simulink library "cordic_rotation_mode"  (R2018b)
settings: Solver=VariableStepAuto  StartTime=0.0  StopTime=10.0  RelTol=1e-3
undefined symbols (not defined in the file or in its folder): nIters
settings Model: Creator=jimjoy  LastModifiedBy=tbryan
settings DataIOCC: ReturnWorkspaceOutputs=on

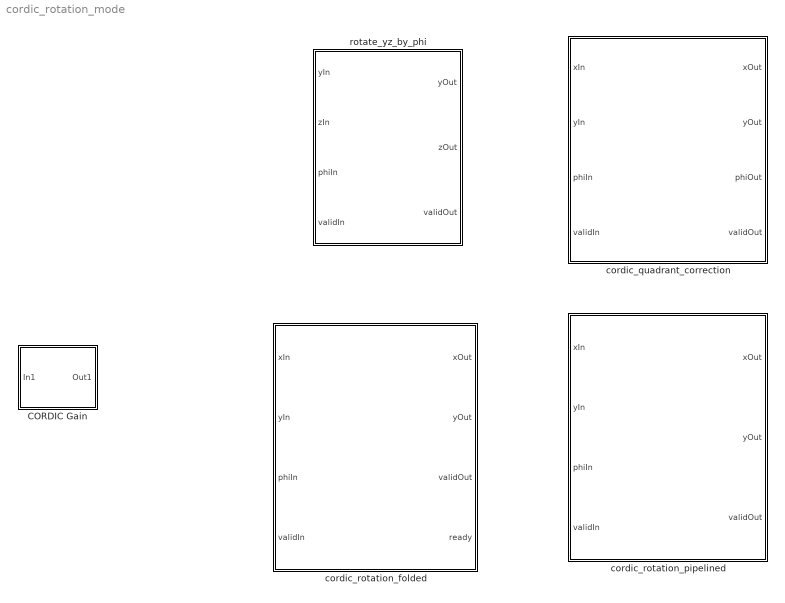
== system cordic_rotation_mode ==
  CORDIC Gain : Subsystem  mask{nIters=nIters}
      mask prompts: nIters "Number of CORDIC Iterations"
  cordic_quadrant_correction : MATLAB Function  TreatAsAtomicUnit=on
  cordic_rotation_folded : MATLAB Function  TreatAsAtomicUnit=on  mask{nIters=nIters}
      mask prompts: nIters "Number of CORDIC Iterations"
  cordic_rotation_pipelined : MATLAB Function  TreatAsAtomicUnit=on
  rotate_yz_by_phi : MATLAB Function  TreatAsAtomicUnit=on  mask{nIters=nIters}
      mask prompts: nIters "Number of CORDIC Iterations"

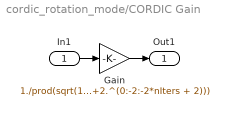
== system cordic_rotation_mode/CORDIC Gain ==
  In1 : Inport
  Gain : Gain  Gain=1./prod(sqrt(1+2.^(0:-2:-2*nIters + 2)))  OutDataTypeStr=Inherit: Same as input
  Out1 : Outport
  wires:
  Gain/1 -> Out1/1
  In1/1 -> Gain/1

== matlab function cordic_rotation_mode/cordic_quadrant_correction ==
  settings: fimath=hdlfimath
  data: xIn input; xOut output; yIn input; phiIn input; validIn input boolean; yOut output; phiOut output; validOut output
function [xOut, yOut, phiOut, validOut] = cordic_quadrant_correction(xIn, yIn, phiIn, validIn)
    
    % Copyright 2018 The MathWorks, Inc.
    %#codegen
   
    persistent xReg yReg phiReg validReg
    
    T = constructTypesTable(xIn, yIn, phiIn, validIn);
    
    if isempty(xReg)
       xReg = cast(0,'like',T.x);
       yReg = cast(0,'like',T.y);
       phiReg = cast(0,'like',T.phi);
       validReg = cast(0,'like',T.validIn);
    end
    
    xOut = xReg;
    yOut = yReg;
    phiOut = phiReg;
    validOut = validReg;
   

    [xReg, yReg, phiReg] = cordicQuadrantCorrectionKernel(xIn, yIn, phiIn, T);
    validReg = cast(validIn, 'like', T.validIn);
    
end

function T = constructTypesTable(x, y ,phi, validIn)
    % This convenience function constructs the types table for the
    % cordic quadrant correction. It also provides some top level
    % assertions that are evaluated at compile time.
    coder.inline('always');
    if isfloat(x)
        assert(isfloat(y),'X and Y must Both be floating poitn values')
        isHDL = coder.target('HDL');
        assert(~isHDL,'Floating-point is not supported for this function in HDL Code Generation');
        T.x = cast([],'like',x);
        T.y = cast([],'like',y);
    elseif isfi(x)
        assert(isfi(y), 'X and Y must both be fi objects');
        assert(isscaledtype(x) && isscaledtype(y),'X and Y must be scaled types');
        % Assert that the wordlength and fraction length are equal
        assert((x.WordLength == y.WordLength) && ...
                              (x.FractionLength == y.FractionLength),'X and Y must have the same word and fraction lengths');
        wl = max(8, x.WordLength);
        fl = min(wl - 3, x.FractionLength);
        F = hdlfimath();
        T.x = fi([],1,wl,fl,F);
        T.y = fi([],1,wl,fl,F);
    else
       assert(false,'Type not supported');
    end
    
    assert(isfloat(phi) || (isfi(phi) && isscaledtype(phi)), 'phi must be either floating point or a scaled fi type');
    T.phi = cast([],'like',phi);
    
    assert(islogical(validIn) || (isfi(validIn) && isboolean(validIn)),'validIn must be logical');
    T.validIn = cast([],'like',validIn);
end

function [xOut, yOut, phiOut] = cordicQuadrantCorrectionKernel(x, y, phi, T)
    coder.inline('always');
    xOut = cast(x,'like',T.x);
    yOut = cast(y,'like',T.y);
    phiOut = cast(phi,'like',T.phi);
    if (phi > coder.const(cast(pi/2,'like', T.phi))) && ...
            (phi < coder.const(cast(1.5*pi,'like', T.phi)))
        phiOut(:) = phi - cast(pi,'like', T.phi);
        xOut(:) = -x;
        yOut(:) = -y;
    elseif (phi > coder.const(cast(1.5*pi,'like', T.phi)))
        phiOut(:) = phi - cast(2*pi,'like', T.phi);
        xOut(:) = x;
        yOut(:) = y;
    elseif (phi < cast(-0.5*pi,'like', T.phi))
        phiOut(:) = phi + cast(pi,'like',T.phi);
        xOut(:) = -x;
        yOut(:) = -y;
    end
end

== matlab function cordic_rotation_mode/rotate_yz_by_phi ==
  settings: fimath=hdlfimath
  data: yIn input; zIn input; yOut output; zOut output; phiIn input; validIn input; validOut output; nIters parameter
function [yOut, zOut, validOut] = rotate_by_phi(yIn, zIn, phiIn, validIn, nIters)
    %#codegen
    
    %Copyright 2018 The MathWorks, Inc.
    
    persistent yReg zReg validReg phiReg
    
    yNumericTypeInternal = numerictype(1,yIn.WordLength + 3, yIn.FractionLength + 3);
    zNumericTypeInternal = numerictype(1,zIn.WordLength + 3, zIn.FractionLength + 3);
    phiNumericTypeInternal = numerictype(1,zIn.WordLength+3, zIn.FractionLength + 3);
    
    if isempty(yReg)
        yReg = fi(zeros(1,nIters+2), yNumericTypeInternal);
        zReg = fi(zeros(1,nIters+2), zNumericTypeInternal);
        phiReg = fi(zeros(1,nIters+2), phiNumericTypeInternal);
        validReg = false(1,nIters+2);
    end
    
    yOut = cast(yReg(end),'like',yIn);
    zOut = cast(zReg(end),'like',zIn);
    validOut = validReg(end);
    coder.unroll
    for ii = nIters+2:-1:1
        if ii == 1
            [yReg(ii), zReg(ii), phiReg(ii), validReg(ii)] = ...
                readInputs(yIn, zIn, phiIn, validIn);
        elseif ii == 2
            validReg(ii) = validReg(ii - 1);
            [yReg(ii), zReg(ii), phiReg(ii)] = ...
                cordicQuadrantCorrection(yReg(ii-1), zReg(ii - 1), phiReg(ii-1));
        else
            validReg(ii) = validReg(ii - 1);
            [yReg(ii), zReg(ii), phiReg(ii)] = ...
                cordicRotationKernel(yReg(ii-1), zReg(ii - 1), phiReg(ii - 1),...
                ii, nIters);
        end
    end
    
end

function [y, z, phi, valid] = readInputs(yIn, zIn, phiIn, validIn)
    y = yIn;
    z = zIn;
    phi = phiIn;
    valid = validIn;
end

function [yOut, zOut, phiOut] = cordicQuadrantCorrection(y, z, phi)
    yOut = y;
    zOut = z;
    phiOut = phi;
    if (phi > coder.const(cast(pi/2,'like',phi))) && ...
            (phi < coder.const(cast(1.5*pi,'like',phi)))
        phiOut(:) = phi - cast(pi,'like',phi);
        yOut(:) = -y;
        zOut(:) = -z;
    elseif (phi > coder.const(cast(1.5*pi,'like',phi)))
        phiOut(:) = phi - cast(2*pi,'like',phi);
        yOut(:) = y;
        zOut(:) = z;
    end
end

function [yOut, zOut, phiOut] = cordicRotationKernel(y, z, phi, iterNum, numIters)
    angleTable = coder.const(getAngleTable(numIters,phi));
    y0 = bitsra(y,iterNum - 3);
    z0 = bitsra(z,iterNum - 3);
    yOut = y;
    zOut = z;
    phiOut = phi;
    if phi > 0
        % Rotate in the positive direction
        yOut(:) = y - z0;
        zOut(:) = z + y0;
        phiOut(:) = phi - angleTable(iterNum - 2);
    else
        % Rotate in the negative direction
        yOut(:) = y + z0;
        zOut(:) = z - y0;
        phiOut(:) = phi + angleTable(iterNum - 2);
    end
end

function angleTable = getAngleTable(numIters, T)
    angleTable = cast(atan(2.^(0:-1:-numIters + 1)),'like',T);
end

== matlab function cordic_rotation_mode/cordic_rotation_pipelined ==
  settings: fimath=hdlfimath
  data: xIn input; xOut output; yIn input; phiIn input; validIn input; yOut output; validOut output; nIters parameter
function [xOut, yOut, validOut] = cordic_rotation_pipelined(xIn, yIn, phiIn, validIn, nIters)
   
    % Copyright 2018 The MathWorks, Inc.
    
    %#codegen
    
    persistent xReg yReg validReg phiReg
    
    T = getTypesTable(xIn, yIn, phiIn, validIn);
    
    if isempty(xReg)
       xReg = zeros(nIters + 1,1,'like',T.x);
       yReg = zeros(nIters + 1,1,'like',T.y);
       phiReg = zeros(nIters + 1,1,'like',T.phi);
       validReg = zeros(nIters + 1,1,'like',T.validIn);
    end
    
    xOut = xReg(end);
    yOut = yReg(end);
    validOut = validReg(end);
    
    validReg(:) = [validIn; validReg(1:end-1)];
    [xReg(2:end), yReg(2:end), phiReg(2:end)] = ...
        cordicRotationKernel(xReg(1:end-1), yReg(1:end-1), phiReg(1:end-1), nIters, T);
    xReg(1) = xIn;
    yReg(1) = yIn;
    phiReg(1) = phiIn;
    
end

function T = getTypesTable(x, y, phi, validIn)
    % This convenience function constructs the types table for the
    % cordic quadrant correction. It also provides some top level
    % assertions that are evaluated at compile time.
    coder.inline('always');
    if isfloat(x)
        assert(isfloat(y),'X and Y must Both be floating poitn values')
        isHDL = coder.target('HDL');
        assert(~isHDL,'Floating-point is not supported for this function in HDL Code Generation');
        T.x = cast([],'like',x);
        T.y = cast([],'like',y);
    elseif isfi(x)
        assert(isfi(y), 'X and Y must both be fi objects');
        assert(isscaledtype(x) && isscaledtype(y),'X and Y must be scaled types');
        % Assert that the wordlength and fraction length are equal
        assert((x.WordLength == y.WordLength) && ...
            (x.FractionLength == y.FractionLength),'X and Y must have the same word and fraction lengths');
        wl = max(8, x.WordLength);
        fl = min(wl - 3, x.FractionLength);
        F = hdlfimath();
        T.x = fi([],1,wl,fl,F);
        T.y = fi([],1,wl,fl,F);
    else
        assert(false,'Type not supported');
    end
    
    assert(isfloat(phi) || (isfi(phi) && isscaledtype(phi)), 'phi must be either floating point or a scaled fi type');
    T.phi = cast([],'like',phi);
    
    assert(islogical(validIn) || (isfi(validIn) && isboolean(validIn)),'validIn must be logical');
    T.validIn = cast([],'like',validIn);
end

function [xOut, yOut, phiOut] = cordicRotationKernel(xIn, yIn, phiIn, nIters, T)
    xOut = zeros(nIters,1,'like',T.x);
    yOut = zeros(nIters,1,'like',T.y);
    phiOut = zeros(nIters,1,'like',T.phi);
    
    angleTable = coder.const(cast(atan(2.^(0:-1:-nIters+1)),'like',T.phi));
    
    for ii = nIters:-1:1
       if phiIn(ii) > 0
           xOut(ii) = xIn(ii) - bitsra(yIn(ii),ii-1);
           yOut(ii) = yIn(ii) + bitsra(xIn(ii),ii-1);
           phiOut(ii) = phiIn(ii) - angleTable(ii);
       else
           xOut(ii) = xIn(ii) + bitsra(yIn(ii),ii-1);
           yOut(ii) = yIn(ii) - bitsra(xIn(ii),ii-1);
           phiOut(ii) = phiIn(ii) + angleTable(ii);
       end
    end
    
end

== matlab function cordic_rotation_mode/cordic_rotation_folded ==
  settings: fimath=hdlfimath
  data: xIn input; xOut output; yIn input; phiIn input; validIn input; yOut output; validOut output boolean; nIters parameter; ready output
function [xOut, yOut, validOut, ready] = cordic_rotation_folded(xIn, yIn, phiIn, validIn, nIters)
    
    % Copyright 2018 The MathWorks, Inc.
    %#codegen

    persistent xReg yReg phiReg validReg iterReg readyReg
    
    T = getTypesTable(xIn, yIn, phiIn, validIn);
    
    xOut = cast(0,'like',T.x);
    yOut = cast(0,'like',T.y);
    validOut = cast(0,'like',T.validIn);
    ready = false;
    
    iterWL = nextpow2(nIters);
    
    if isempty(xReg)
        xReg = cast(0,'like',T.x);
        yReg = cast(0,'like',T.y);
        phiReg = cast(0,'like',T.phi);
        validReg = cast(0,'like',T.validIn);
        iterReg = fi(0,0,iterWL, 0, hdlfimath);
        readyReg = true;
    end
    
    xOut(:) = xReg;
    yOut(:) = yReg;
    validOut(:) = validReg;
    ready(:) = readyReg;
    
    if iterReg == 0
        xReg(:) = xIn;
        yReg(:) = yIn;
        phiReg(:) = phiIn;
        validReg(:) = false;
        if validIn
            iterReg(:) = iterReg + 1;
            readyReg(:) = false;
        else
            iterReg(:) = 0;
            readyReg(:) = true;
        end
    elseif (iterReg < nIters) 
        [xReg, yReg, phiReg] = cordicRotationKernel(xReg, yReg, phiReg, iterReg, T, nIters);
        iterReg(:) = iterReg + 1;
        validReg(:) = false;
        readyReg(:) = false;
    elseif iterReg == nIters
        [xReg, yReg, phiReg] = cordicRotationKernel(xReg, yReg, phiReg, iterReg, T, nIters);
        iterReg(:) = 0;
        validReg(:) = true;
        readyReg(:) = true;
    else
        xReg(:) = xIn;
        yReg(:) = yIn;
        phiReg(:) = phiIn;
        validReg(:) = false;
        readyReg(:) = readyReg;
    end  
end

function T = getTypesTable(x, y, phi, validIn)
    % This convenience function constructs the types table for the
    % cordic quadrant correction. It also provides some top level
    % assertions that are evaluated at compile time.
    coder.inline('always');
    if isfloat(x)
        assert(isfloat(y),'X and Y must Both be floating poitn values')
        isHDL = coder.target('HDL');
        assert(~isHDL,'Floating-point is not supported for this function in HDL Code Generation');
        T.x = cast([],'like',x);
        T.y = cast([],'like',y);
    elseif isfi(x)
        assert(isfi(y), 'X and Y must both be fi objects');
        assert(isscaledtype(x) && isscaledtype(y),'X and Y must be scaled types');
        % Assert that the wordlength and fraction length are equal
        assert((x.WordLength == y.WordLength) && ...
            (x.FractionLength == y.FractionLength),'X and Y must have the same word and fraction lengths');
        wl = max(8, x.WordLength);
        fl = min(wl - 3, x.FractionLength);
        F = hdlfimath();
        T.x = fi([],1,wl,fl,F);
        T.y = fi([],1,wl,fl,F);
    else
        assert(false,'Type not supported');
    end
    
    assert(isfloat(phi) || (isfi(phi) && isscaledtype(phi)), 'phi must be either floating point or a scaled fi type');
    T.phi = cast([],'like',phi);
    
    assert(islogical(validIn) || (isfi(validIn) && isboolean(validIn)),'validIn must be logical');
    T.validIn = cast([],'like',validIn);
end

function [xOut, yOut, phiOut] = cordicRotationKernel(x, y, phi, iterNum, T, nIters)
    angleTable = coder.const(cast(atan(2.^(0:-1:-nIters+1)),'like',T.phi));
    x0 = bitsra(x, iterNum - 1);
    y0 = bitsra(y, iterNum - 1);
    xOut = cast(0,'like',T.x);
    yOut = cast(0,'like',T.y);
    phiOut = cast(0,'like',T.phi);
    if phi < 0
        xOut(:) = x + y0;
        yOut(:) = y - x0;
        phiOut(:) = phi + angleTable(iterNum);
    else
        xOut(:) = x - y0;
        yOut(:) = y + x0;
        phiOut(:) = phi - angleTable(iterNum);
    end
end
